simulink model "SVPWM_inverter"  (R2024b)
settings: Solver=VariableStepAuto  StartTime=0.0  StopTime=1  FixedStep=1e-6  MaxStep=1e-5  RelTol=1e-4
undefined symbols (not defined in the file): Down, GPTRIP1SEL, TZ1, Up
libraries: spsIGBTDiodeLib x6, spsCurrentMeasurementLib x3, spsVoltageMeasurementLib x3, spsDCVoltageSourceLib x1, spsGroundLib x1, simulink x1, c2802xlib x1, spsTHDLib x1, spsThreePhaseSeriesRLCBranchLib x1, spspowerguiLib x1
settings Model: Creator=ahmed  LastModifiedBy=ahmed

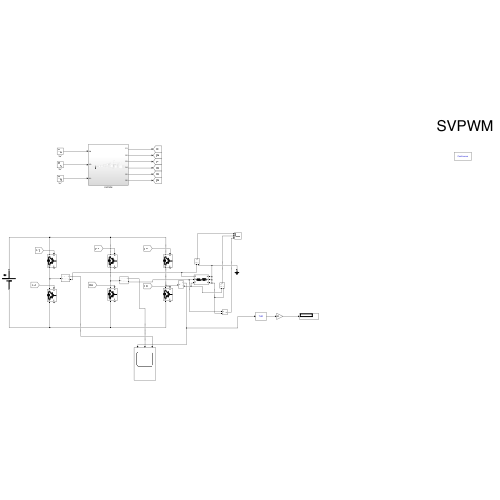
[thumbnail: Simulink's stored preview of the top-level diagram]
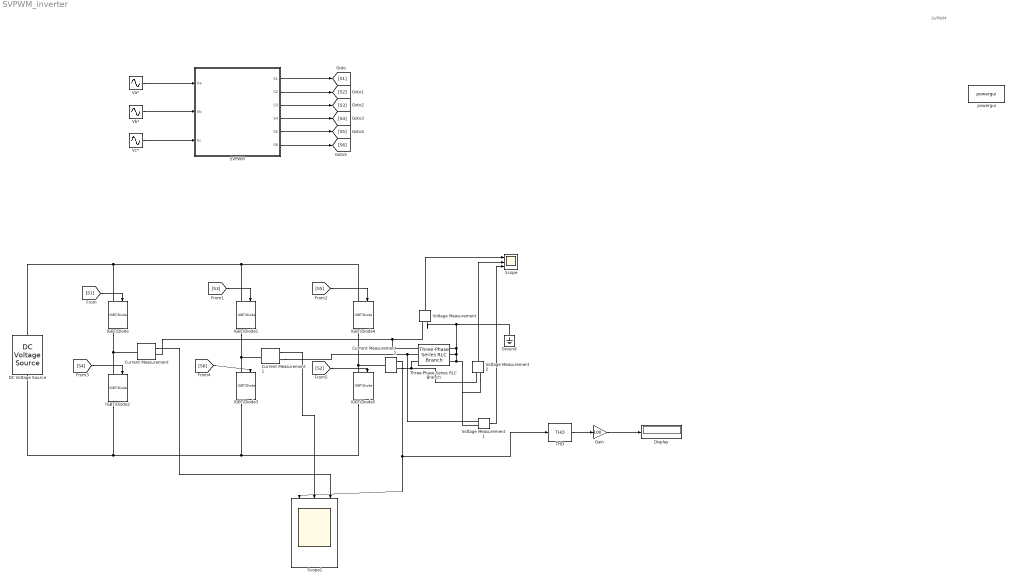
== system SVPWM_inverter ==
  note: SVPWM
  Current Measurement : spsCurrentMeasurementLib/Current Measurement  PhasorSimulation=off  OutputType=Complex  PSBequivalent=0
  Current Measurement1 : spsCurrentMeasurementLib/Current Measurement  PhasorSimulation=off  OutputType=Complex  PSBequivalent=0
  Current Measurement2 : spsCurrentMeasurementLib/Current Measurement  PhasorSimulation=off  OutputType=Complex  PSBequivalent=0
  DC Voltage Source : spsDCVoltageSourceLib/DC Voltage Source  Amplitude=320  Measurements=None
  Display : Display
  Gain : Gain  Gain=100
  Ground : spsGroundLib/Ground  LConnTagsString=a
  IGBT/Diode{,1..5} (6 alike) : spsIGBTDiodeLib/IGBT//Diode  Ron=1e-3  Rs=1e5  Cs=inf  Measurements=on
  SVPWM : Subsystem
  Scope : Scope  NumInputPorts=3
  Scope1 : Scope  NumInputPorts=3
  THD : spsTHDLib/THD  Freq=50  Ts=0
  Three-Phase Series RLC Branch : spsThreePhaseSeriesRLCBranchLib/Three-Phase Series RLC Branch  LConnTagsString=A|B|C  RConnTagsString=A|B|C  BranchType=RL  Resistance=20  Inductance=20e-3  Capacitance=0  Measurements=None
  Va* : Sin  Amplitude=220*sqrt(2)*.97/sqrt(3)  Frequency=2*pi*50  SampleTime=0
  Vb* : Sin  Amplitude=220*sqrt(2)*.97/sqrt(3)  Frequency=2*pi*50  Phase=-(2*pi/3)  SampleTime=0
  Vc* : Sin  Amplitude=220*sqrt(2)*.97/sqrt(3)  Frequency=2*pi*50  Phase=2*pi/3  SampleTime=0
  Voltage Measurement : spsVoltageMeasurementLib/Voltage Measurement  PhasorSimulation=off  OutputType=Complex  PSBequivalent=0
  Voltage Measurement1 : spsVoltageMeasurementLib/Voltage Measurement  PhasorSimulation=off  OutputType=Complex  PSBequivalent=0
  Voltage Measurement2 : spsVoltageMeasurementLib/Voltage Measurement  PhasorSimulation=off  OutputType=Complex  PSBequivalent=0
  powergui : spspowerguiLib/powergui  Priority=1  SimulationMode=Continuous  SampleTime=50e-6  frequency=60  Iterations=50  frequencyindice=0  Pbase=100e6  ErrMax=1e-4  UnitsV=kV  UnitsW=MW  buscounter=0  FunctionMessages=off  echomessages=off  EnableUseOfTLC=off  CurrentSourceSwitches=off  DisableSnubberDevices=off  DisableRonSwitches=off  DisableVfSwitches=off  DisplayEquations=off  AutomaticDiscreteSolvers=off  SolverType=Tustin/Backward Euler (TBE)  Interpol=off  ExternalGateDelay=off  methode=off  Ts=100  x0status=blocks  SPID=on  SwTol=0  HookPort=off  NonlinearTolerance=1e-4  nMaxIteration=100  ContinueOnMaxIteration=off  RestoreLinks=warning  ResistiveCurrentMeasurement=off  Frange=[0:2:500]  Ylog=off  Xlog=on  ShowGrid=off  save=off  variable=ZData  structure=0  ZoomFFT=off  StartTime=0.0  cycles=1  DisplayStyle=1  fundamental=60  FreqAxis=off  MaxFrequency=1000  frequencyindicesteady=1  RmsSteady=1  display=off
  wires:
  Va*/1 -> SVPWM/1(Va)
  Vc*/1 -> SVPWM/3(Vc)
  Vb*/1 -> SVPWM/2(Vb)
  SVPWM/1(S1) -> [S1]
  SVPWM/2(S2) -> [S2]
  SVPWM/3(S3) -> [S3]
  SVPWM/4(S4) -> [S4]
  SVPWM/5(S5) -> [S5]
  SVPWM/6(S6) -> [S6]
  [S1] -> IGBT/Diode/1
  [S3] -> IGBT/Diode1/1
  [S5] -> IGBT/Diode4/1
  [S4] -> IGBT/Diode2/1
  [S6] -> IGBT/Diode3/1
  [S2] -> IGBT/Diode5/1
  Voltage Measurement/1 -> Scope/1
  Voltage Measurement2/1 -> Scope/2
  Voltage Measurement1/1 -> Scope/3
  Current Measurement2/1 -> THD/1, Scope1/1
  Current Measurement1/1 -> Scope1/2
  Current Measurement/1 -> Scope1/3
  THD/1 -> Gain/1
  Gain/1 -> Display/1
  connections:
  IGBT/Diode4/LConn1 -- IGBT/Diode1/LConn1 -- IGBT/Diode/LConn1 -- DC Voltage Source/RConn1
  IGBT/Diode5/RConn1 -- IGBT/Diode3/RConn1 -- IGBT/Diode2/RConn1 -- DC Voltage Source/LConn1
  IGBT/Diode4/RConn1 -- Current Measurement2/LConn1 -- IGBT/Diode5/LConn1
  IGBT/Diode1/RConn1 -- Current Measurement1/LConn1 -- IGBT/Diode3/LConn1
  IGBT/Diode/RConn1 -- Current Measurement/LConn1 -- IGBT/Diode2/LConn1
  Three-Phase Series RLC Branch/RConn1 -- Voltage Measurement1/LConn2 -- Voltage Measurement2/LConn2 -- Three-Phase Series RLC Branch/RConn3 -- Three-Phase Series RLC Branch/RConn2 -- Ground/LConn1 -- Voltage Measurement/LConn2
  Three-Phase Series RLC Branch/LConn1 -- Current Measurement/RConn1 -- Voltage Measurement/LConn1
  Three-Phase Series RLC Branch/LConn2 -- Current Measurement1/RConn1 -- Voltage Measurement1/LConn1
  Three-Phase Series RLC Branch/LConn3 -- Current Measurement2/RConn1 -- Voltage Measurement2/LConn1

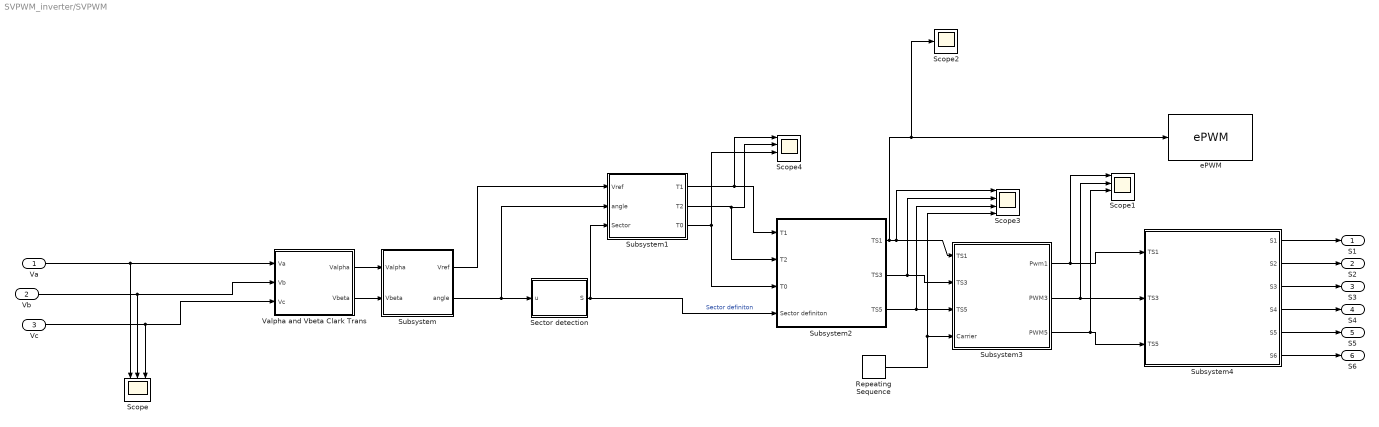
== system SVPWM_inverter/SVPWM ==
  Va : Inport
  Vb : Inport  Port=2
  Vc : Inport  Port=3
  Repeating Sequence : simulink/Sources/Repeating Sequence  rep_seq_t=[0 1/30000 1/15000]  rep_seq_y=[0 1/15000 0]
  Scope : Scope  NumInputPorts=3
  Scope1 : Scope  NumInputPorts=4
  Scope2 : Scope
  Scope3 : Scope  NumInputPorts=4
  Scope4 : Scope  NumInputPorts=4
  Sector detection : MATLAB Function  TreatAsAtomicUnit=on
  Subsystem : Subsystem
  Subsystem1 : Subsystem
  Subsystem2 : Subsystem
  Subsystem3 : Subsystem
  Subsystem4 : Subsystem
  Valpha and Vbeta Clark Trans : Subsystem
  ePWM : c2802xlib/ePWM  PwmType=C2000_Type4  useModule=ePWM1  ePWMxLINKTBPRD=Not Linked  periodUnits=Clock cycles  timerSource=Specify via dialog  timerPeriod_clk=64000  timerPeriod_sec=0.0001  tbshadow=Counter equals to zero  countingMode=Up-Down  phaseActiveEnable=Disable  phaseDirection=Count down after sync  phaseActive=0  synchronizationEnable=off  dcaevt1Sync=off  dcbevt1Sync=off  synchronizationOption=Disable  dcbevt1SyncOut=off  dcaevt1SyncOut=off  cmpdSyncOut=off  cmpcSyncOut=off  cmpbSyncOut=off  zeroSyncOut=off  swfSyncOut=off  perSynchronizationOption=Counter equals to period (CTR=PRD)  clockPrescale=1  HSclockPrescale=1  enswap=off  ePWMxAStatus=on  ePWMxAactionLogic1=Do nothing  ePWMxAactionLogic2=Do nothing  ePWMxAactionLogic3=Clear  ePWMxAactionLogic4=Set  ePWMxAactionLogic5=Do nothing  ePWMxAactionLogic6=Do nothing  ePWMxACSFenable=off  ePWMxACSFvalue=Forcing disable  ePWMxASFreload=Zero  ePWMxBStatus=on  ePWMxBactionLogic1=Do nothing  ePWMxBactionLogic2=Do nothing  ePWMxBactionLogic3=Set  ePWMxBactionLogic4=Clear  ePWMxBactionLogic5=Do nothing  ePWMxBactionLogic6=Do nothing  ePWMxBCSFenable=off  ePWMxBCSFvalue=Forcing disable  ePWMxBSFreload=Zero  ePWNxBOutWay=off  ePWMxLINKCMPA=Not Linked  CMPAUnits=Percentages  CMPASource=Input port  CMPAValue_per=0  CMPAValue_clk=32000  enCMPAshadow=Counter equals to zero (CTR=Zero)  ePWMxLINKCMPB=Not Linked  CMPBUnits=Clock cycles  CMPBSource=Specify via dialog  CMPBValue_per=50  CMPBValue_clk=32000  enCMPBshadow=Counter equals to zero (CTR=Zero)  ePWMxLINKCMPC=Not Linked  CMPCUnits=Clock cycles  CMPCSource=Specify via dialog  CMPCValue_per=50  CMPCValue_clk=32000  enCMPCshadow=Counter equals to zero (CTR=Zero)  ePWMxLINKCMPD=Not Linked  CMPDUnits=Clock cycles  CMPDSource=Specify via dialog  CMPDValue_per=50  CMPDValue_clk=32000  enCMPDshadow=Counter equals to zero (CTR=Zero)  enableDBePWMxA=on  enableDBePWMxB=on  enhalfcycle=off  DBpolarity=Active high complementary (AHC)  DBedgeDelay=Positive  DBSource_ePWMxA=ePWMxA  DBSource_ePWMxB=ePWMxA  DBPeriodUnits=Seconds  DBperiodSource=Specify via dialog  REDperiod=0  FEDperiod=0  REDperiod_sec=1e-6  FEDperiod_sec=1e-6  LoadModeDBRED=Immediate without using shadow  LoadModeDBFED=Immediate without using shadow  adcstartModuleA=off  adcrequestEventA=First event  adcstartEventA=Digital Compare Module A Event 1 start of conversion (DCAEVT1.soc)  adcstartEventA_type2=Counter equals to zero (CTR=Zero)  adcstartModuleB=off  adcrequestEventB=First event  adcstartEventB=Counter equals to zero (CTR=Zero)  adcstartEventB_type2=Counter equals to zero (CTR=Zero)  intEn=off  intPrd=First event  intSel=Counter equals to zero (CTR=Zero)  intSel_type2=Counter equals to zero (CTR=Zero)  hrpe=off  enHRPWM=off  HRPWM_LoadMode=Counter equals to period (CTR=PRD)  HRPWM_CTLMode=Duty or Period control mode  HRPWM_EDGMode=Both edge  hrpeb=off  enHRPWMB=off  HRPWM_LoadModeB=Counter equals to zero (CTR=ZERO)  HRPWM_CTLModeB=Duty or Period control mode  HRPWM_EDGModeB=Both edge  enHRDBRED=off  enHRDBFED=off  enSFO=on  enautoconv=on  chopperEnable=off  chopperFrequency=1  chopperFirstwidth=1  chopperDuty=12.5%  tripZonesource=Specify via dialog  tzselOSHT1=off  tzselOSHT2=off  tzselOSHT3=off  tzselOSHT4=off  tzselOSHT5=off  tzselOSHT6=off  tzselOSHDCAEV1=off  tzselOSHDCBEV1=off  tzselCBC1=off  tzselCBC2=off  tzselCBC3=off  tzselCBC4=off  tzselCBC5=off  tzselCBC6=off  tzselCBCDCAEV2=off  tzselCBCDCBEV2=off  enTzOstIntr=off  enTzCbcIntr=off  enTzDCAEVT1Intr=off  enTzDCAEVT2Intr=off  enTzDCBEVT1Intr=off  enTzDCBEVT2Intr=off  tzclrCBCLatch=Counter equals to zero (CTR=Zero)  ePWMxAforced=No action  ePWMxBforced=No action  DCAEVT1forced=No action  DCBEVT1forced=No action  DCAEVT2forced=No action  DCBEVT2forced=No action  dcah=Trip Zone 1 input (TZ1)  dcal=Trip Zone 2 input (TZ2)  dcbh=Trip Zone 1 input (TZ1)  dcbl=Trip Zone 2 input (TZ2)  dcah_type2=GPTRIP1SEL/(TZ1)  dcal_type2=GPTRIP1SEL/(TZ1)  dcbh_type2=GPTRIP1SEL/(TZ1)  dcbl_type2=GPTRIP1SEL/(TZ1)  gendcaevt1=Event disabled  gendcaevt2=Event disabled  gendcbevt1=Event disabled  gendcbevt2=Event disabled  dcaevt1src=DCAEVT1 with sync  dcaevt2src=DCAEVT2 with sync  dcbevt1src=DCBEVT1 with sync  dcbevt2src=DCBEVT2 with sync  pulsesel=Counter equals to zero (CTR=Zero)  blankinv=off  blankoffset=0  blankwidth=0  evsrcsel=Filtered version of DCAEVT1 (DCAEVT1FILT)  encape=off
      settings: LibrarySourceBlock=c2837xDlib/ePWM
  S1 : Outport
  S2 : Outport  Port=2
  S3 : Outport  Port=3
  S4 : Outport  Port=4
  S5 : Outport  Port=5
  S6 : Outport  Port=6
  wires:
  Subsystem4/5(S5) -> S5/1
  Sector detection/1(S) -> Subsystem2/4(Sector definiton), Subsystem1/3(Sector)  "Sector definiton"
  Subsystem/2(angle) -> Sector detection/1(u), Subsystem1/2(angle)
  Subsystem/1(Vref) -> Subsystem1/1(Vref)
  Valpha and Vbeta Clark Trans/2(Vbeta) -> Subsystem/2(Vbeta)
  Va/1 -> Valpha and Vbeta Clark Trans/1(Va), Scope/1
  Repeating Sequence/1 -> Scope3/4, Subsystem3/4(Carrier)
  Valpha and Vbeta Clark Trans/1(Valpha) -> Subsystem/1(Valpha)
  Vb/1 -> Valpha and Vbeta Clark Trans/2(Vb), Scope/2
  Vc/1 -> Valpha and Vbeta Clark Trans/3(Vc), Scope/3
  Subsystem1/2(T2) -> Scope4/2, Subsystem2/2(T2)
  Subsystem1/1(T1) -> Scope4/1, Subsystem2/1(T1)
  Subsystem1/3(T0) -> Subsystem2/3(T0), Scope4/3
  Subsystem2/1(TS1) -> Scope2/1, ePWM/1, Subsystem3/1(TS1), Scope3/1
  Subsystem2/2(TS3) -> Subsystem3/2(TS3), Scope3/2
  Subsystem2/3(TS5) -> Subsystem3/3(TS5), Scope3/3
  Subsystem3/1(Pwm1) -> Scope1/1, Subsystem4/1(TS1)
  Subsystem3/2(PWM3) -> Scope1/2, Subsystem4/2(TS3)
  Subsystem3/3(PWM5) -> Scope1/3, Subsystem4/3(TS5)
  Subsystem4/1(S1) -> S1/1
  Subsystem4/2(S2) -> S2/1
  Subsystem4/3(S3) -> S3/1
  Subsystem4/4(S4) -> S4/1
  Subsystem4/6(S6) -> S6/1

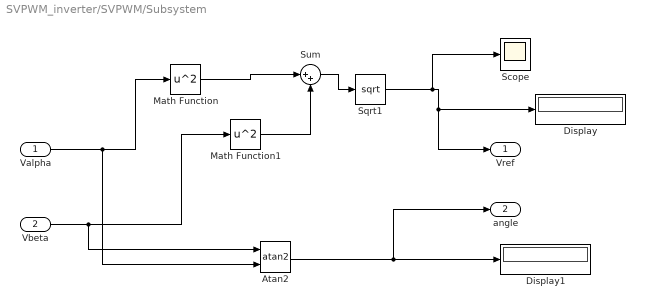
== system SVPWM_inverter/SVPWM/Subsystem ==
  Valpha : Inport
  Vbeta : Inport  Port=2
  Atan2 : Trigonometry  Operator=atan2
  Display : Display
  Display1 : Display
  Math Function : Math  Operator=square
  Math Function1 : Math  Operator=square
  Scope : Scope
  Sqrt1 : Sqrt
  Sum : Sum  Inputs=|++
  Vref : Outport
  angle : Outport  Port=2
  wires:
  Valpha/1 -> Atan2/2, Math Function/1
  Vbeta/1 -> Atan2/1, Math Function1/1
  Math Function/1 -> Sum/1
  Math Function1/1 -> Sum/2
  Sum/1 -> Sqrt1/1
  Sqrt1/1 -> Scope/1, Vref/1, Display/1
  Atan2/1 -> Display1/1, angle/1

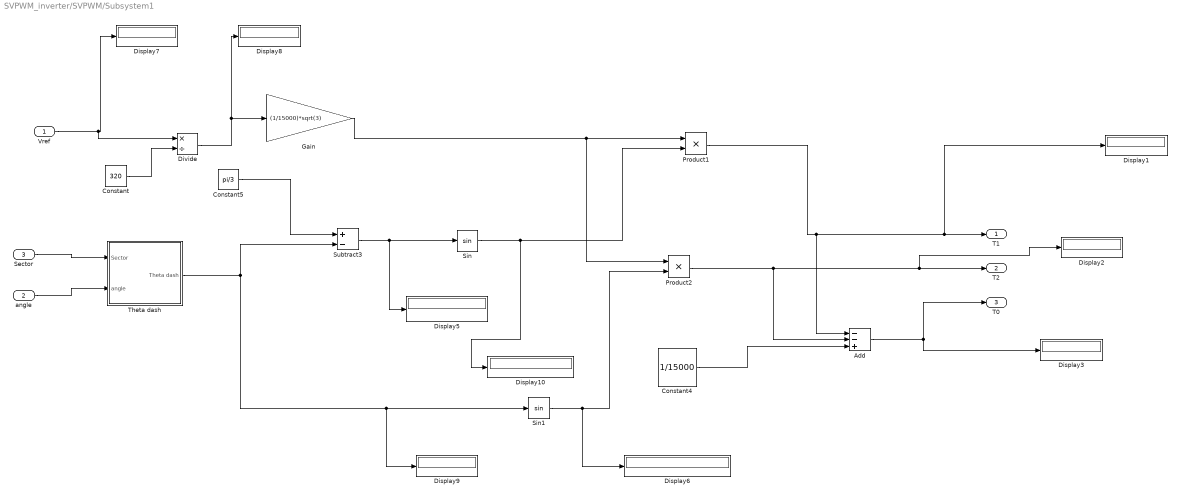
== system SVPWM_inverter/SVPWM/Subsystem1 ==
  Vref : Inport
  angle : Inport  Port=2
  Sector : Inport  Port=3
  Add : Sum  Inputs=--+
  Constant : Constant  Value=320
  Constant4 : Constant  Value=1/15000
  Constant5 : Constant  Value=pi/3
  Display{1..3,5..10} (9 alike) : Display
  Divide : Product  Inputs=*/
  Gain : Gain  Gain=(1/15000)*sqrt(3)
  Product1 : Product
  Product2 : Product
  Sin : Trigonometry
  Sin1 : Trigonometry
  Subtract3 : Sum  Inputs=+-
  Theta dash : Subsystem
  T1 : Outport
  T2 : Outport  Port=2
  T0 : Outport  Port=3
  wires:
  Gain/1 -> Product2/1, Product1/1
  Product1/1 -> Display1/1, T1/1, Add/1
  Sin1/1 -> Display6/1, Product2/2
  Product2/1 -> Add/2, Display2/1, T2/1
  Constant4/1 -> Add/3
  Add/1 -> Display3/1, T0/1
  Constant5/1 -> Subtract3/1
  Subtract3/1 -> Sin/1, Display5/1
  Sin/1 -> Display10/1, Product1/2
  Divide/1 -> Display8/1, Gain/1
  Sector/1 -> Theta dash/1(Sector)
  angle/1 -> Theta dash/2(angle)
  Theta dash/1(Theta dash) -> Display9/1, Sin1/1, Subtract3/2
  Constant/1 -> Divide/2
  Vref/1 -> Divide/1, Display7/1

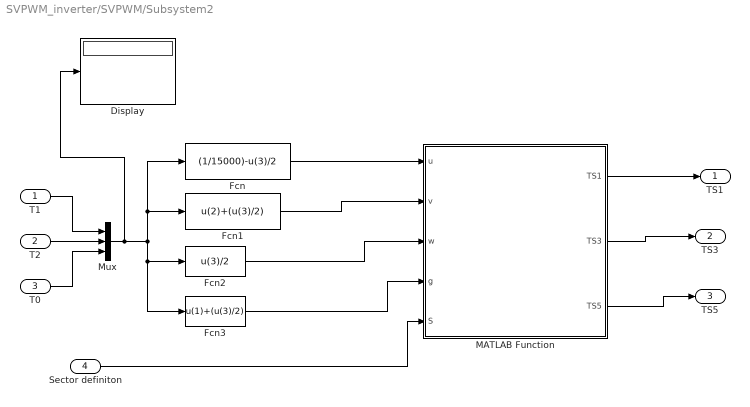
== system SVPWM_inverter/SVPWM/Subsystem2 ==
  T1 : Inport
  T2 : Inport  Port=2
  T0 : Inport  Port=3
  Sector definiton : Inport  Port=4
  Display : Display
  Fcn : Fcn  Expr=(1/15000)-u(3)/2
  Fcn1 : Fcn  Expr=u(2)+(u(3)/2)
  Fcn2 : Fcn  Expr=u(3)/2
  Fcn3 : Fcn  Expr=u(1)+(u(3)/2)
  MATLAB Function : MATLAB Function  TreatAsAtomicUnit=on
  Mux : Mux  Inputs=3
  TS1 : Outport
  TS3 : Outport  Port=2
  TS5 : Outport  Port=3
  wires:
  MATLAB Function/1(TS1) -> TS1/1
  MATLAB Function/3(TS5) -> TS5/1
  MATLAB Function/2(TS3) -> TS3/1
  T1/1 -> Mux/1
  T2/1 -> Mux/2
  T0/1 -> Mux/3
  Mux/1 -> Display/1, Fcn1/1, Fcn/1, Fcn3/1, Fcn2/1
  Fcn/1 -> MATLAB Function/1(u)
  Fcn1/1 -> MATLAB Function/2(v)
  Fcn2/1 -> MATLAB Function/3(w)
  Fcn3/1 -> MATLAB Function/4(g)
  Sector definiton/1 -> MATLAB Function/5(S)

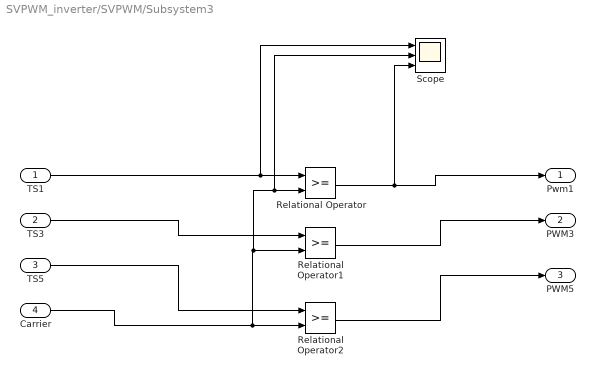
== system SVPWM_inverter/SVPWM/Subsystem3 ==
  TS1 : Inport
  TS3 : Inport  Port=2
  TS5 : Inport  Port=3
  Carrier : Inport  Port=4
  Relational Operator : RelationalOperator  OutDataTypeStr=boolean  RndMeth=Simplest  InputSameDT=off
  Relational Operator1 : RelationalOperator  OutDataTypeStr=boolean  RndMeth=Simplest  InputSameDT=off
  Relational Operator2 : RelationalOperator  OutDataTypeStr=boolean  RndMeth=Simplest  InputSameDT=off
  Scope : Scope  NumInputPorts=3
  Pwm1 : Outport
  PWM3 : Outport  Port=2
  PWM5 : Outport  Port=3
  wires:
  TS1/1 -> Scope/1, Relational Operator/1
  TS3/1 -> Relational Operator1/1
  TS5/1 -> Relational Operator2/1
  Carrier/1 -> Scope/2, Relational Operator/2, Relational Operator1/2, Relational Operator2/2
  Relational Operator/1 -> Scope/3, Pwm1/1
  Relational Operator1/1 -> PWM3/1
  Relational Operator2/1 -> PWM5/1

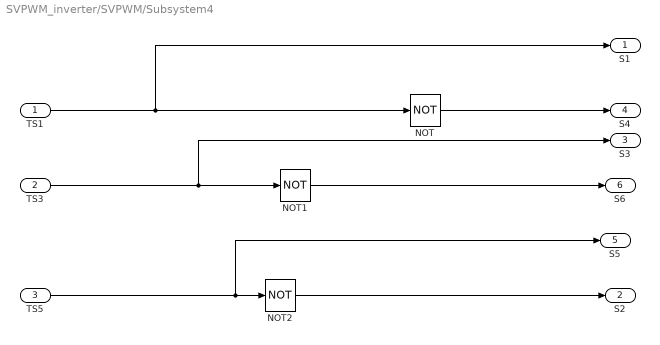
== system SVPWM_inverter/SVPWM/Subsystem4 ==
  TS1 : Inport
  TS3 : Inport  Port=2
  TS5 : Inport  Port=3
  NOT : Logic  Operator=NOT  IconShape=distinctive  AllPortsSameDT=off  OutDataTypeStr=boolean
  NOT1 : Logic  Operator=NOT  IconShape=distinctive  AllPortsSameDT=off  OutDataTypeStr=boolean
  NOT2 : Logic  Operator=NOT  IconShape=distinctive  AllPortsSameDT=off  OutDataTypeStr=boolean
  S1 : Outport
  S2 : Outport  Port=2
  S3 : Outport  Port=3
  S4 : Outport  Port=4
  S5 : Outport  Port=5
  S6 : Outport  Port=6
  wires:
  NOT2/1 -> S2/1
  TS5/1 -> NOT2/1, S5/1
  NOT1/1 -> S6/1
  TS3/1 -> S3/1, NOT1/1
  NOT/1 -> S4/1
  TS1/1 -> S1/1, NOT/1

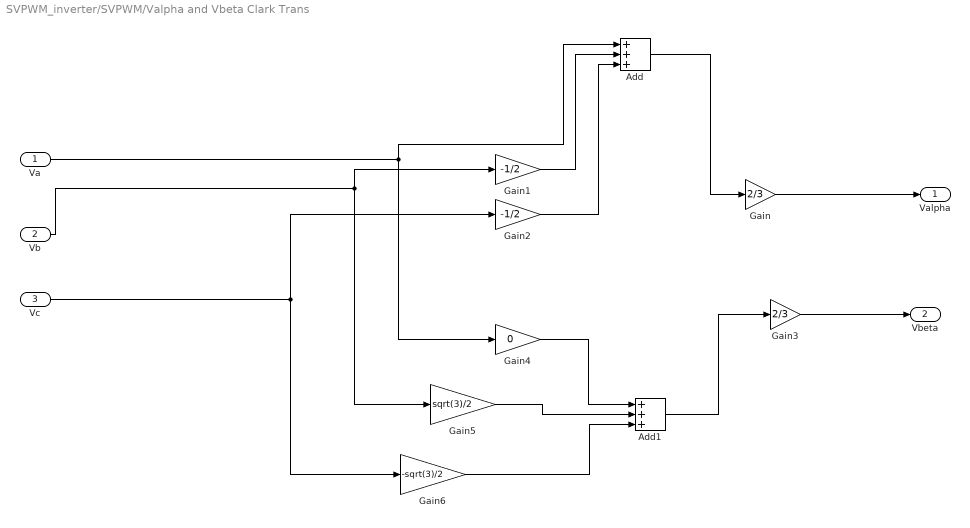
== system SVPWM_inverter/SVPWM/Valpha and Vbeta Clark Trans ==
  Va : Inport
  Vb : Inport  Port=2
  Vc : Inport  Port=3
  Add : Sum  Inputs=+++
  Add1 : Sum  Inputs=+++
  Gain : Gain  Gain=2/3
  Gain1 : Gain  Gain=-1/2
  Gain2 : Gain  Gain=-1/2
  Gain3 : Gain  Gain=2/3
  Gain4 : Gain  Gain=0
  Gain5 : Gain  Gain=sqrt(3)/2
  Gain6 : Gain  Gain=-sqrt(3)/2
  Valpha : Outport
  Vbeta : Outport  Port=2
  wires:
  Va/1 -> Add/1, Gain4/1
  Vb/1 -> Gain5/1, Gain1/1
  Gain1/1 -> Add/2
  Vc/1 -> Gain2/1, Gain6/1
  Gain2/1 -> Add/3
  Add/1 -> Gain/1
  Gain4/1 -> Add1/1
  Gain5/1 -> Add1/2
  Gain6/1 -> Add1/3
  Add1/1 -> Gain3/1
  Gain/1 -> Valpha/1
  Gain3/1 -> Vbeta/1

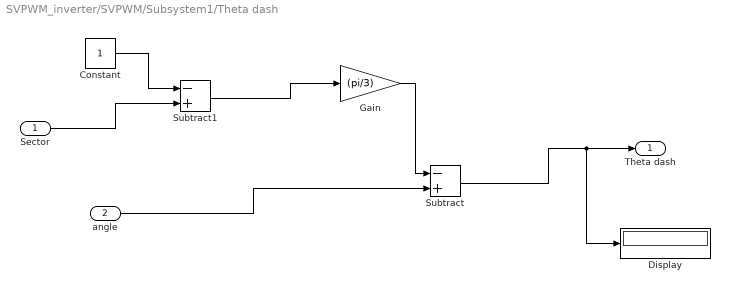
== system SVPWM_inverter/SVPWM/Subsystem1/Theta dash ==
  Sector : Inport
  angle : Inport  Port=2
  Constant : Constant
  Display : Display
  Gain : Gain  Gain=(pi/3)
  Subtract : Sum  Inputs=-+
  Subtract1 : Sum  Inputs=-+
  Theta dash : Outport
  wires:
  angle/1 -> Subtract/2
  Gain/1 -> Subtract/1
  Constant/1 -> Subtract1/1
  Sector/1 -> Subtract1/2
  Subtract1/1 -> Gain/1
  Subtract/1 -> Display/1, Theta dash/1

== matlab function SVPWM_inverter/SVPWM/Subsystem2/MATLAB Function ==
  data: TS1 output; u input; TS3 output; TS5 output; v input; w input; g input; S input
function [TS1, TS3,TS5] = fcn(u, v, w, g,S)

switch S
    case 1
        TS1 = u;
        TS3 = v;
        TS5 = w;
    case 2
        TS1 = g;
        TS3 = u;
        TS5 = w;
    case 3
        TS1 = w;
        TS3 = u;
        TS5 = v;
    case 4
        TS1 = w;
        TS3 = g;
        TS5 = u;
    case 5
        TS1 = v;
        TS3 = w;
        TS5 = u;
    case 6
        TS1 = u;
        TS3 = w;
        TS5 = g;
    otherwise
      TS1=0;  
      TS3=0;  
      TS5=0; 
end
end

== matlab function SVPWM_inverter/SVPWM/Sector detection ==
  data: u input; S output
function S = fcn(u)

u = (180/pi)* u;

if(u < 60 && u >= 0)
    u = 1;
elseif(u < 120 && u >= 60)
    u = 2;
elseif(u < 180 && u >= 120)
    u = 3;
elseif(u < -120 && u >= -180)
u = 4;
elseif(u < -60 && u >= -120)
u = 5;
elseif(u < 0 && u >= -60)
u = 6;
else
    u = 0;
end
S = u;
